simulink subsystem "Combustion_Model"  (R2020b)
settings: Solver=VariableStepAuto  StartTime=0.0  StopTime=10.0  RelTol=1e-3
model mask{useOxidiserFluxOnlyRegRateEquation=0}
  mask prompts: useOxidiserFluxOnlyRegRateEquation "Use oxidiser flux only regression rate equation?"
undefined symbols (not defined in the file): grainOuterDiam, Sim
settings Model: Creator=Edward  LastModifiedBy=Edward

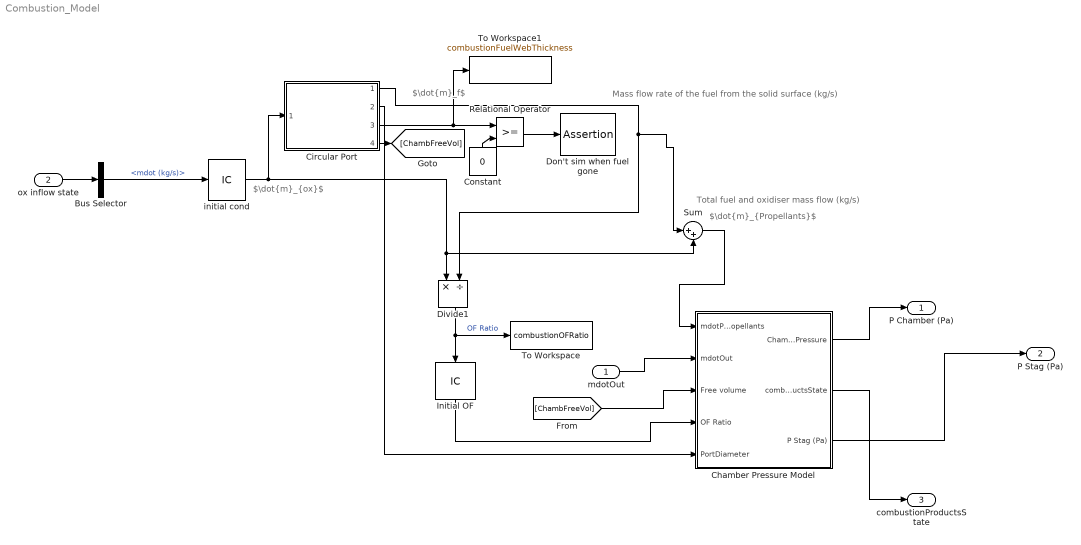
== system Combustion_Model ==
  note: $\dot{m}_f$
  note: $\dot{m}_{ox}$
  note: $\dot{m}_{Propellants}$
  note: Total fuel and oxidiser mass flow (kg/s)
  note: Mass flow rate of the fuel from the solid surface (kg/s)
  mdotOut : Inport
  ox inflow state : Inport  Port=2
  Bus Selector : BusSelector  OutputSignals=mdot (kg/s)
  Chamber Pressure Model : Subsystem
  Circular Port : Subsystem  ReferencedSubsystem=Circular_Port_Model
  Constant : Constant  Value=0
  Divide1 : Product  Inputs=*/
  Don't sim when fuel gone : Assertion
  "Initial OF " : InitialCondition  Value=Sim.combustionChamber.OFRatioInitial
  Relational Operator : RelationalOperator  OutDataTypeStr=boolean  RndMeth=Simplest
  Sum : Sum  Inputs=|++
  To Workspace : ToWorkspace  VariableName=combustionOFRatio  SaveFormat=Timeseries  SampleTime=-1
  To Workspace1 : ToWorkspace  VariableName=combustionFuelWebThickness  SaveFormat=Timeseries  SampleTime=-1
  initial cond : InitialCondition  Value=Sim.combustionChamber.mdotOxInitial
  P Chamber (Pa) : Outport
  "P Stag (Pa) " : Outport  Port=2
  combustionProductsState : Outport  Port=3
  wires:
  Circular Port/2 -> Chamber Pressure Model/5(PortDiameter)
  Chamber Pressure Model/3("P Stag (Pa) ") -> "P Stag (Pa) "/1
  mdotOut/1 -> Chamber Pressure Model/2(mdotOut)
  Chamber Pressure Model/1(Chamber Pressure) -> P Chamber (Pa)/1
  Sum/1 -> Chamber Pressure Model/1(mdotPropellants)
  Circular Port/3 -> Relational Operator/1, To Workspace1/1
  Constant/1 -> Relational Operator/2
  Relational Operator/1 -> Don't sim when fuel gone/1
  Circular Port/1 -> Sum/1, Divide1/2
  "Initial OF "/1 -> Chamber Pressure Model/4(OF Ratio)
  initial cond/1 -> Divide1/1, Sum/2, Circular Port/1
  Divide1/1 -> "Initial OF "/1, To Workspace/1  "OF Ratio"
  Circular Port/4 -> [ChambFreeVol]
  [ChambFreeVol] -> Chamber Pressure Model/3(Free volume)
  ox inflow state/1 -> Bus Selector/1
  Bus Selector/1 -> initial cond/1  "<mdot (kg/s)>"
  Chamber Pressure Model/2(combustionProductsState) -> combustionProductsState/1

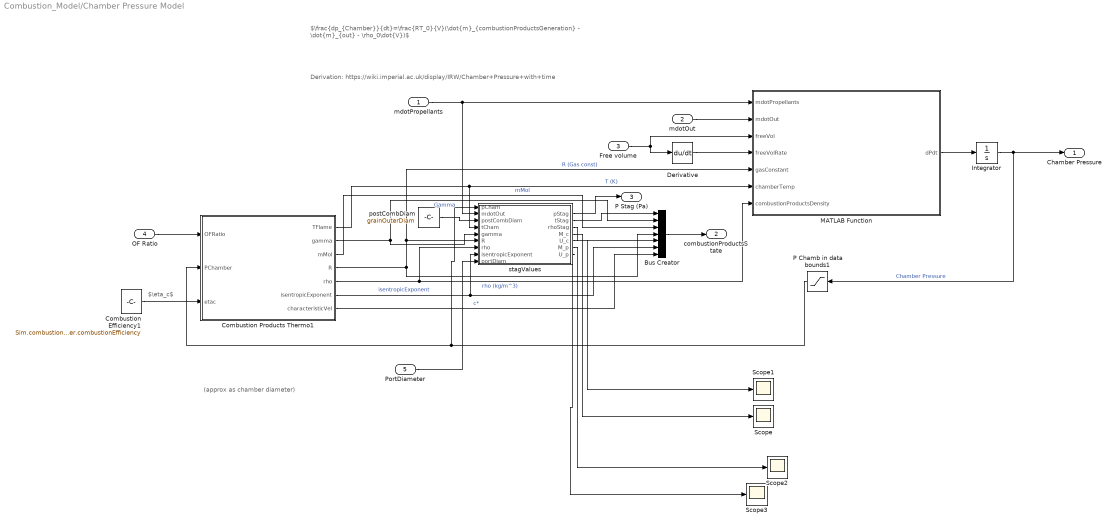
== system Combustion_Model/Chamber Pressure Model ==
  note: $\eta_c$
  note: $\frac{dp_{Chamber}}{dt}=\frac{RT_0}{V}(\dot{m}_{combustionProductsGeneration} - \dot{m}_{out} - \rho_0\dot{V})$
  note: Derivation: https://wiki.imperial.ac.uk/display/IRW/Chamber+Pressure+with+time
  note: (approx as chamber diameter)
  mdotPropellants : Inport
  mdotOut : Inport  Port=2
  Free volume : Inport  Port=3
  OF Ratio : Inport  Port=4
  PortDiameter : Inport  Port=5
  Bus Creator : BusCreator  Inputs=7
  Combustion Efficiency1 : Constant  Value=Sim.combustionChamber.combustionEfficiency
  Combustion Products Thermo1 : MATLAB Function  TreatAsAtomicUnit=on
  Derivative : Derivative
  Integrator : Integrator  InitialCondition=Sim.combustionChamber.PChamberInit
  MATLAB Function : MATLAB Function  TreatAsAtomicUnit=on
  P Chamb in data bounds1 : Saturate  UpperLimit=Sim.combustionChamber.artificalPChamberMax  LowerLimit=50000
  Scope{,1..3} (4 alike) : Scope
  postCombDiam : Constant  Value=grainOuterDiam
  stagValues : MATLAB Function  TreatAsAtomicUnit=on
  Chamber Pressure : Outport
  combustionProductsState : Outport  Port=2
  "P Stag (Pa) " : Outport  Port=3
  wires:
  Bus Creator/1 -> combustionProductsState/1
  mdotPropellants/1 -> stagValues/2(mdotOut), MATLAB Function/1(mdotPropellants)
  Free volume/1 -> MATLAB Function/3(freeVol), Derivative/1
  Combustion Products Thermo1/5(rho) -> stagValues/7(rho), MATLAB Function/7(combustionProductsDensity)  "rho (kg/m^3)"
  Combustion Products Thermo1/1(TFlame) -> stagValues/4(tCham), MATLAB Function/6(chamberTemp)  "T (K)"
  Combustion Products Thermo1/4(R) -> Bus Creator/4, stagValues/6(R), MATLAB Function/5(gasConstant)  "R (Gas const)"
  Combustion Efficiency1/1 -> Combustion Products Thermo1/3(etac)
  OF Ratio/1 -> Combustion Products Thermo1/1(OFRatio)
  Derivative/1 -> MATLAB Function/4(freeVolRate)
  mdotOut/1 -> MATLAB Function/2(mdotOut)
  MATLAB Function/1(dPdt) -> Integrator/1
  Integrator/1 -> P Chamb in data bounds1/1, Chamber Pressure/1  "Chamber Pressure"
  P Chamb in data bounds1/1 -> stagValues/1(pCham), Combustion Products Thermo1/2(PChamber)
  stagValues/1(pStag) -> "P Stag (Pa) "/1
  Combustion Products Thermo1/7(characteristicVel) -> Bus Creator/7  "c*"
  Combustion Products Thermo1/6(isentropicExponent) -> stagValues/8(isentropicExponent), Bus Creator/6  "isentropicExponent"
  stagValues/3(rhoStag) -> Bus Creator/5
  Combustion Products Thermo1/3(mMol) -> Bus Creator/3  "mMol"
  postCombDiam/1 -> stagValues/3(postCombDiam)
  Combustion Products Thermo1/2(gamma) -> Bus Creator/2, stagValues/5(gamma)  "Gamma"
  stagValues/2(tStag) -> Bus Creator/1
  stagValues/4(M_c) -> Scope/1
  stagValues/5(U_c) -> Scope1/1
  stagValues/7(U_p) -> Scope3/1
  stagValues/6(M_p) -> Scope2/1
  PortDiameter/1 -> stagValues/9(portDiam)

== matlab function Combustion_Model/Chamber Pressure Model/MATLAB Function ==
  data: mdotPropellants input; dPdt output; mdotOut input; freeVol input; freeVolRate input; gasConstant input; chamberTemp input; combustionProductsDensity input
function dPdt = chamberPressureRate(mdotPropellants, mdotOut, ...
    freeVol, freeVolRate, gasConstant, chamberTemp, combustionProductsDensity)
%Unsteady combustion chamber pressure
%
%Inputs:
%mdotPropellants = Rate of combustion products generation (kg/s)
%mdotOut = Rate of combustion products leaving chamber (kg/s)
%freeVol = Instantaneous free volume in the chamber (m^3)
%freeVolRate = Time rate of change of freeVol (m^3/s)
%gasConstant = Gas specific constant (Eg. 287 for air) of combustion
%products
%chamberTemp = Temp of combustion chamber, often taken to be adiabatic
%flame temp (K)
%combustionProductsDensity = Density of combustion products (kg/m^3)
%
%Assumptions:
%-Relationship between pressure change rate and density change rate given
%by ideal gas law
%-Similar derivation to: http://www.nakka-rocketry.net/th_pres.html#Pressure
dPdt = ((gasConstant.*chamberTemp)./freeVol) .* (mdotPropellants - mdotOut - combustionProductsDensity.*freeVolRate);

== matlab function Combustion_Model/Chamber Pressure Model/Combustion Products Thermo1 ==
  data: OFRatio input; TFlame output; PChamber input; etac input; gamma output; mMol output; R output; rho output; isentropicExponent output; characteristicVel output; propepProps parameter
function [TFlame, gamma, mMol, R, rho, isentropicExponent, characteristicVel] = combustionProductsProperties(OFRatio, PChamber, etac, propepProps)
%Keep within data. TODO: Expand dataset
if(OFRatio > 10)
   OFRatio = 10; 
end
if(OFRatio < 2.003)
   OFRatio = 2.003; 
end
[TFlame, gamma, mMol, R, rho, isentropicExponent, characteristicVel] = HybridMotor.chamberDataInterp(propepProps, OFRatio, PChamber, etac);
%Assume ideal gas:
%P = rho*R*T -> rho = P/(R*T)

== matlab function Combustion_Model/Chamber Pressure Model/stagValues ==
  data: pCham input; mdotOut input; postCombDiam input; pStag output; tCham input; tStag output; rhoStag output; M_c output; U_c output; gamma input; R input; rho input; isentropicExponent input; portDiam input; M_p output; U_p output
function [pStag,tStag,rhoStag,M_c,U_c,M_p,U_p] = stagValues(pCham,mdotOut,postCombDiam,tCham,gamma,R,rho,isentropicExponent,portDiam)
A_p = portDiam^2/4*pi;
A_c = postCombDiam^2/4*pi;
U_p = mdotOut/A_p/rho; %flow speed in port (incompressible)
U_c = mdotOut/A_c/rho; %flow speed in postComb (incompressible)

a = sqrt(gamma*R*tCham); %speed of sound in postComb
M_p = U_p/a; %mach number in port
M_c = U_c/a; %mach number in postComb
tStag = tCham*(1+(isentropicExponent-1)/2*M_c^2); %stagnation temp
pStag = pCham*(1+(isentropicExponent-1)/2*M_c^2)^(isentropicExponent/(isentropicExponent-1)); %stag pressure
rhoStag = pCham*(1+(isentropicExponent-1)/2*M_c^2)^(1/(isentropicExponent-1)); %stag density

end
